simulink model "Speed_Controller_Test_gr2"  (Simulink 7.0)
settings: Solver=ode4  SolverMode=SingleTasking  StartTime=0.0  StopTime=252  FixedStep=0.01  RelTol=1e-3
InitFcn:
  | tempomat_para
StopFcn:
  | clear;
values from neighbouring files (symbols this model uses):
  A = 1.9    [tempomat_para.m]
  a_Fzg_max = 2    [tempomat_para.m]
  a_Fzg_min = -2    [tempomat_para.m]
  cw = 0.32    [tempomat_para.m]
  gang = [1 2 3 4]    [tempomat_para.m]
  gang_vec = [1 2 3 4]    [tempomat_para.m]
  i_anteil = 5    [tempomat_para.m]
  i_d = 3.42    [tempomat_para.m]
  i_g = [3.91 2.17 1.37 1.00]    [tempomat_para.m]
  lambda_gang = [1.3 1.25  1.17  1.05]    [tempomat_para.m]
  m_Fzg = 1400    [tempomat_para.m]
  M_mot_max = [130 149 163 170 168 166 162 158 150 139 123 80]    [tempomat_para.m]
  M_mot_min = [0 -40]    [tempomat_para.m]
  n_mot0 = 1000    [tempomat_para.m]
  n_mot_max = 1000:500:6500    [tempomat_para.m]
  n_mot_min = [1000 6500]    [tempomat_para.m]
  p_anteil = 100    [tempomat_para.m]
  r_dyn = 0.28    [tempomat_para.m]
  rho = 1.202    [tempomat_para.m]
  t_sch = 0.2    [tempomat_para.m]
  TI = [block '/TI']    [PSTI_callback.m]
  v_Fzg_ms0 = 0    [tempomat_para.m]
undefined symbols (not defined in the file or in its folder): Drossel_mat, getdatatypespecs
libraries: simulink x116, fzgbib x3
(part 1 of 10)
settings Model: Creator=Abel  LastModifiedBy=jza
settings DataIOCC: LimitDataPoints=off  SignalLoggingName=sigsOut
settings OptimizationCC: BooleanDataType=off
settings DebuggingCC: SaveWithParameterizedLinksMsg=none  SignalResolutionControl=TryResolveAllWithWarning  InheritedTsInSrcMsg=none  MultiTaskDSMMsg=warning  MultiTaskCondExecSysMsg=none  StrictBusMsg=None
settings RTWCC: IncludeERTFirstTime=on
settings GRTTargetCC: TargetFcnLib=ansi_tfl_tmw.mat

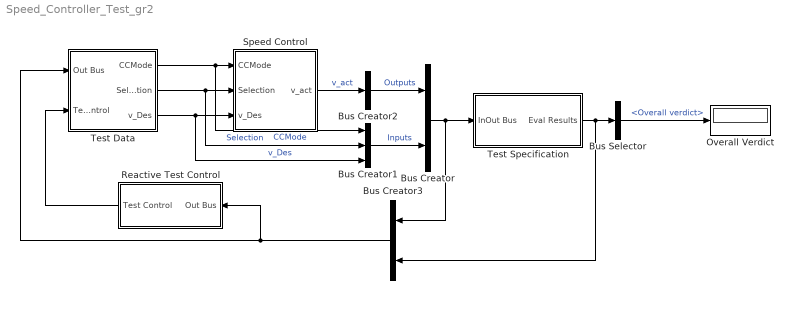
== system Speed_Controller_Test_gr2 ==
  Bus Creator : BusCreator  Inputs=2
  Bus Creator1 : BusCreator  Inputs=3
  Bus Creator2 : BusCreator  Inputs=1
  Bus Creator3 : BusCreator  Orientation=left  Inputs=2
  Bus Selector : BusSelector  OutputSignals=Overall verdict
  Overall Verdict : Display
  Reactive Test Control : Subsystem  Orientation=left
  Speed Control : Subsystem
  Test Data : Subsystem
  Test Specification : Subsystem  Description=Test evaluation system template. Create a new test evaluation system from this template.
  wires:
  Speed Control/1(v_act) -> Bus Creator2/1  "v_act"
  Bus Creator/1 -> Test Specification/1(InOut Bus), Bus Creator3/1
  Bus Creator2/1 -> Bus Creator/1  "Outputs"
  Bus Creator1/1 -> Bus Creator/2  "Inputs"
  Test Data/3(v_Des) -> Speed Control/3(v_Des), Bus Creator1/3  "v_Des"
  Bus Creator3/1 -> Test Data/1(Out Bus), Reactive Test Control/1(Out Bus)
  Test Specification/1(Eval Results) -> Bus Creator3/2, Bus Selector/1
  Reactive Test Control/1(Test Control) -> Test Data/2(Test Control)
  Bus Selector/1 -> Overall Verdict/1  "<Overall verdict>"
  Test Data/1(CCMode) -> Speed Control/1(CCMode), Bus Creator1/1  "CCMode"
  Test Data/2(Selection) -> Speed Control/2(Selection), Bus Creator1/2  "Selection"

== system Speed_Controller_Test_gr2/Reactive Test Control ==
  Out Bus : Inport  OutDataType=sfix(16)  OutScaling=2^0
  Bus Selector : BusSelector  OutputSignals=signal2.signal1.signal1.signal1.signal1.Local verdict
  Counter : Subsystem
  Memory : Memory
  OR : Logic  Operator=OR  Inputs=3  AllPortsSameDT=off  OutDataTypeMode=boolean
  Switch : Switch  Criteria=u2 > Threshold
  error : simulink/Logic and Bit Operations/Compare To Constant  SystemSampleTime=-1  relop===  const=-1  LogicOutDataTypeMode=uint8  ZeroCross=off
  fail : simulink/Logic and Bit Operations/Compare To Constant  SystemSampleTime=-1  relop===  const=0  LogicOutDataTypeMode=uint8  ZeroCross=off
  pass : simulink/Logic and Bit Operations/Compare To Constant  SystemSampleTime=-1  relop===  const=1  LogicOutDataTypeMode=uint8  ZeroCross=off
  test case 1 : Constant  OutDataType=sfix(16)  OutScaling=2^0
  test case 2 : Constant  Value=2  OutDataType=sfix(16)  OutScaling=2^0
  Test Control : Outport  OutDataType=sfix(16)  OutScaling=2^0
  wires:
  OR/1 -> Counter/1(In1), Counter/Trigger
  test case 1/1 -> Switch/3
  Out Bus/1 -> Bus Selector/1
  Switch/1 -> Test Control/1
  test case 2/1 -> Switch/1
  Counter/1(Out1) -> Switch/2
  Bus Selector/1 -> Memory/1  "<Local verdict>"
  pass/1 -> OR/1
  fail/1 -> OR/2
  error/1 -> OR/3
  Memory/1 -> pass/1, error/1, fail/1

== system Speed_Controller_Test_gr2/Speed Control ==
  CCMode : Inport  OutDataType=sfix(16)  OutScaling=2^0
  Selection : Inport  Port=2  OutDataType=sfix(16)  OutScaling=2^0
  v_Des : Inport  Port=3  OutDataType=sfix(16)  OutScaling=2^0
  " Speed Controller " : Subsystem  AncestorBlock=fzgbib/GeschwindigkeitsRegelung
  Terminator1 : Terminator
  Terminator2 : Terminator
  Vehicle Model : Subsystem
      mask Type: Vehicle Model
      mask Display: image(imread('car.jpg','jpg'),[0.05,0.2,0.9,0.6])
  v_act : Outport  OutDataType=sfix(16)  OutScaling=2^0
  wires:
  Vehicle Model/2(M_Br_b) -> Terminator1/1
  Vehicle Model/3(M_Mot_b) -> Terminator2/1
  " Speed Controller "/1(CarInputs) -> Vehicle Model/1(StellgroessenTempomat)
  Vehicle Model/1(FzgDaten) -> " Speed Controller "/1(CarOutputs)
  " Speed Controller "/2(v_act) -> v_act/1
  v_Des/1 -> " Speed Controller "/2(CCMode)
  Selection/1 -> " Speed Controller "/3(Selection)
  CCMode/1 -> " Speed Controller "/4(v_Des)

== system Speed_Controller_Test_gr2/Test Data ==
  Out Bus : Inport  OutDataType=sfix(16)  OutScaling=2^0
  Test Control : Inport  Port=2  OutDataType=sfix(16)  OutScaling=2^0
  Bus Creator : BusCreator  Inputs=6
  Bus Selector : BusSelector  OutputSignals=v_Des (signal 1),v_Des (signal 4)
  Bus Selector1 : BusSelector  OutputSignals=CCMode (signal 2),CCMode (signal 5)
  Bus Selector2 : BusSelector  OutputSignals=Selection (signal 3),Selection (signal 6)
  PrecAct CCMode : MultiPortSwitch  Inputs=3  zeroidx=on
  PrecAct Selection : MultiPortSwitch  Inputs=3  zeroidx=on
  PrecAct v_Des : MultiPortSwitch  Inputs=3  zeroidx=on
  R1 Speed Control step response : Subsystem
  R2 Speed Control velocity restoration time after simple  acceleration/deceleration : Subsystem
  zero signal : Constant  Value=0  OutDataType=sfix(16)  OutScaling=2^0
  CCMode : Outport  OutDataType=sfix(16)  OutScaling=2^0
  Selection : Outport  Port=2  OutDataType=sfix(16)  OutScaling=2^0
  v_Des : Outport  Port=3  OutDataType=sfix(16)  OutScaling=2^0
  wires:
  Out Bus/1 -> R1 Speed Control step response/1(Out Bus)
  PrecAct v_Des/1 -> v_Des/1
  zero signal/1 -> PrecAct v_Des/2, PrecAct Selection/2, PrecAct CCMode/2
  PrecAct CCMode/1 -> CCMode/1
  PrecAct Selection/1 -> Selection/1
  Bus Creator/1 -> Bus Selector/1, Bus Selector1/1, Bus Selector2/1
  Bus Selector/1 -> PrecAct v_Des/3  "<v_Des (signal 1)>"
  R1 Speed Control step response/1(v_Des) -> Bus Creator/1
  R1 Speed Control step response/2(CCMode) -> Bus Creator/2
  R1 Speed Control step response/3(Selection) -> Bus Creator/3
  R2 Speed Control velocity restoration time after simple  acceleration/deceleration/1(v_Des) -> Bus Creator/4
  R2 Speed Control velocity restoration time after simple  acceleration/deceleration/2(CCMode) -> Bus Creator/5
  R2 Speed Control velocity restoration time after simple  acceleration/deceleration/3(Selection) -> Bus Creator/6
  Bus Selector/2 -> PrecAct v_Des/4  "<v_Des (signal 4)>"
  Bus Selector1/1 -> PrecAct CCMode/3  "<CCMode (signal 2)>"
  Bus Selector1/2 -> PrecAct CCMode/4  "<CCMode (signal 5)>"
  Bus Selector2/1 -> PrecAct Selection/3  "<Selection (signal 3)>"
  Bus Selector2/2 -> PrecAct Selection/4  "<Selection (signal 6)>"
  Test Control/1 -> PrecAct v_Des/1, PrecAct CCMode/1, PrecAct Selection/1

== system Speed_Controller_Test_gr2/Test Specification ==
  InOut Bus : Inport  OutDataType=sfix(16)  OutScaling=2^0
  Arbitration : Subsystem
  Bus Creator1 : BusCreator  Inputs=2
  Bus Creator2 : BusCreator  Inputs=2
  Bus Selector1 : BusSelector  OutputSignals=signal1.signal1.signal1.Local verdict,signal1.signal1.signal2.Local verdict,signal2.signal1.signal1.Local verdict
  R1 Speed Control step response : Subsystem  Description=Requirement template. Create a new requirement from this template.
  R2 Speed Control velocity restoration time after simple  acceleration/deceleration : Subsystem  Description=Requirement template. Create a new requirement from this template.
  Signal Conversion : SignalConversion  ConversionOutput=Bus copy
  Eval Results : Outport  OutDataType=sfix(16)  OutScaling=2^0
  wires:
  Signal Conversion/1 -> R1 Speed Control step response/1(InOut Bus), R2 Speed Control velocity restoration time after simple  acceleration/deceleration/1(InOut Bus)
  R1 Speed Control step response/1(Test Info) -> Bus Creator2/1
  InOut Bus/1 -> Signal Conversion/1
  Bus Creator2/1 -> Bus Selector1/1, Bus Creator1/1
  R2 Speed Control velocity restoration time after simple  acceleration/deceleration/1(Test Info) -> Bus Creator2/2
  Bus Selector1/1 -> Arbitration/1(In1)  "<Local verdict>"
  Bus Selector1/2 -> Arbitration/2(In2)  "<Local verdict>"
  Bus Selector1/3 -> Arbitration/3(In3)  "<Local verdict>"
  Bus Creator1/1 -> Eval Results/1
  Arbitration/1(Out1) -> Bus Creator1/2  "Overall verdict"

== system Speed_Controller_Test_gr2/Reactive Test Control/Counter ==
  In1 : Inport  OutDataType=sfix(16)  OutScaling=2^0
  Trigger : TriggerPort
  " 1" : DataTypeConversion  Orientation=down  OutDataType=sfix(16)  OutScaling=2^0
  Add : Sum  OutDataType=sfix(16)  OutScaling=2^-10
  Memory : Memory  Orientation=left  InheritSampleTime=on
  Number of triggers : Constant  Value=2  OutDataType=sfix(16)  OutScaling=2^0
  Relational Operator1 : RelationalOperator  Operator===  LogicOutDataTypeMode=boolean
  Scope1 : Scope  NumInputPorts=4
      settings: YMin=182.932~-5~-5~-5  YMax=202.188~5~5~5  SaveName=ScopeData14  MaxDataPoints=5000000
  Out1 : Outport  OutDataType=sfix(16)  OutScaling=2^0
  wires:
  In1/1 -> Add/1, Scope1/2
  Number of triggers/1 -> Relational Operator1/2
  Relational Operator1/1 -> Out1/1
  Add/1 -> " 1"/1, Relational Operator1/1, Scope1/3
  Memory/1 -> Add/2
  " 1"/1 -> Memory/1

== system Speed_Controller_Test_gr2/Speed Control/ Speed Controller  ==
  CarOutputs : Inport  OutDataType=sfix(16)  OutScaling=2^0
  CCMode : Inport  Port=2  OutDataType=sfix(16)  OutScaling=2^0
  Selection : Inport  Port=3  OutDataType=sfix(16)  OutScaling=2^0
  v_Des : Inport  Port=4  OutDataType=sfix(16)  OutScaling=2^0
  Bus Selector : BusSelector  OutputSignals=i_Total,n_Eng,a_Vhcl,v_act
  Compute SUC inputs : Subsystem  AncestorBlock=fzgbib/StellgroessenBerechnung BeschleunigungsBegrenzung
  Speed Controller : Subsystem  AncestorBlock=fzgbib/GeschwindigkeitsRegelung
  "km/h -> m/s2" : Gain  Gain=1/3.6  ParameterDataType=sfix(16)  ParameterScaling=2^0  OutDataType=sfix(16)  OutScaling=2^0  SaturateOnIntegerOverflow=on
  "m/s2 -> km/h" : Gain  Gain=3.6  ParameterDataType=sfix(16)  ParameterScaling=2^0  OutDataType=sfix(16)  OutScaling=2^0  SaturateOnIntegerOverflow=on
  CarInputs : Outport  OutDataType=sfix(16)  OutScaling=2^0
  v_act : Outport  Port=2  OutDataType=sfix(16)  OutScaling=2^0
  wires:
  Speed Controller/1(T) -> Compute SUC inputs/4(T)
  Bus Selector/1 -> Compute SUC inputs/1(i_Total)  "<i_Total>"
  Bus Selector/2 -> Compute SUC inputs/2(n_Eng)  "<n_Eng>"
  Bus Selector/3 -> Compute SUC inputs/3(a_Vhcl)  "<a_Vhcl>"
  Bus Selector/4 -> Speed Controller/1(v_Vhcl), "m/s2 -> km/h"/1  "<v_act>"
  Compute SUC inputs/1(SUC inputs) -> CarInputs/1
  v_Des/1 -> "km/h -> m/s2"/1
  "km/h -> m/s2"/1 -> Speed Controller/2(v_Des)
  Selection/1 -> Speed Controller/3(Selection)
  CCMode/1 -> Speed Controller/4(CCMode)
  CarOutputs/1 -> Bus Selector/1
  "m/s2 -> km/h"/1 -> v_act/1

== system Speed_Controller_Test_gr2/Speed Control/Vehicle Model ==
  note: i_Gesamt
      | n_mot
      | a_Fzg_mss
      | v_Fzg_ms
      | Gang_i
  StellgroessenTempomat : Inport  Orientation=left  OutDataType=sfix(16)  OutScaling=2^0
  Bremsmomenten beschaenkung : fzgbib/Bremsmomenten beschraenkung  Orientation=left  SystemSampleTime=-1
  Bus Creator : BusCreator  Orientation=left  Inputs=5
  Const : Constant  OutDataType=sfix(16)  OutScaling=2^0
  Fahrzeugmodell : Subsystem  Orientation=left  AncestorBlock=fzgbib/Fahrzeugmodell
  Gangberechnung : fzgbib/Gangberechnung  Orientation=left  SystemSampleTime=-1
  M_Mot M_Br : Demux  Orientation=left  Outputs=2
  Motormoment beschraenkung : fzgbib/Motormoment beschraenkung  Orientation=left  SystemSampleTime=-1
  SG-Koordinator : Subsystem  Orientation=left
  Terminator : Terminator
  FzgDaten : Outport  Orientation=left  OutDataType=sfix(16)  OutScaling=2^0
  M_Br_b : Outport  Orientation=left  Port=2  OutDataType=sfix(16)  OutScaling=2^0
  M_Mot_b : Outport  Orientation=left  Port=3  OutDataType=sfix(16)  OutScaling=2^0
  wires:
  M_Mot M_Br/1 -> Gangberechnung/1, Motormoment beschraenkung/1
  Fahrzeugmodell/5(a_Fzg_mss) -> Bus Creator/3  "a_Vhcl"
  Fahrzeugmodell/1(v_Fzg_ms) -> Bus Creator/4  "v_act"
  Motormoment beschraenkung/1 -> Fahrzeugmodell/2(M_Mot_b), M_Mot_b/1
  M_Mot M_Br/2 -> Bremsmomenten beschaenkung/1
  Fahrzeugmodell/4(Gang_i) -> Gangberechnung/3, Bus Creator/5  "Gang_i"
  Fahrzeugmodell/6("DK_Stellung ") -> Terminator/1
  Fahrzeugmodell/3(n_Mot) -> Gangberechnung/2, Motormoment beschraenkung/2, Bus Creator/2  "n_Eng"
  Fahrzeugmodell/2(i_gesamt) -> Bus Creator/1  "i_Total"
  Gangberechnung/1 -> Fahrzeugmodell/3(Gang_w)
  SG-Koordinator/1(Momente) -> M_Mot M_Br/1
  Bremsmomenten beschaenkung/1 -> Fahrzeugmodell/1(M_Br_b), M_Br_b/1
  StellgroessenTempomat/1 -> SG-Koordinator/1(Tempomat), SG-Koordinator/3(Fahrer)
  Const/1 -> SG-Koordinator/2(TempomatFlag)
  Bus Creator/1 -> FzgDaten/1

== system Speed_Controller_Test_gr2/Test Data/R1 Speed Control step response ==
  Out Bus : Inport  OutDataType=sfix(16)  OutScaling=2^0
  Complete step & CC active + no target & Speed Control active : Subsystem  Description=Preconditions template. Create new preconditions blocks using this template.
  v_Des : Outport  OutDataType=sfix(16)  OutScaling=2^0
  CCMode : Outport  Port=2  OutDataType=sfix(16)  OutScaling=2^0
  Selection : Outport  Port=3  OutDataType=sfix(16)  OutScaling=2^0
  wires:
  Complete step & CC active + no target & Speed Control active/1(v_Des) -> v_Des/1  "v_Des"
  Complete step & CC active + no target & Speed Control active/2(CCMode) -> CCMode/1  "CCMode"
  Complete step & CC active + no target & Speed Control active/3(Selection) -> Selection/1  "Selection"
  Out Bus/1 -> Complete step & CC active + no target & Speed Control active/1(Out Bus)

== system Speed_Controller_Test_gr2/Test Data/R2 Speed Control velocity restoration time after simple  acceleration/deceleration ==
  " CC active + no target & Speed Control active & V_Des increases/decreases  7 times by 1 unit" : Subsystem  Description=Preconditions template. Create new preconditions blocks using this template.
  v_Des : Outport  OutDataType=sfix(16)  OutScaling=2^0
  CCMode : Outport  Port=2  OutDataType=sfix(16)  OutScaling=2^0
  Selection : Outport  Port=3  OutDataType=sfix(16)  OutScaling=2^0
  wires:
  " CC active + no target & Speed Control active & V_Des increases/decreases  7 times by 1 unit"/2(CCMode) -> CCMode/1  "CCMode"
  " CC active + no target & Speed Control active & V_Des increases/decreases  7 times by 1 unit"/3(Selection) -> Selection/1  "Selection"
  " CC active + no target & Speed Control active & V_Des increases/decreases  7 times by 1 unit"/1(v_Des) -> v_Des/1  "v_Des"

== system Speed_Controller_Test_gr2/Test Specification/Arbitration ==
  In1 : Inport  OutDataType=sfix(16)  OutScaling=2^0
  In2 : Inport  Port=2  OutDataType=sfix(16)  OutScaling=2^0
  In3 : Inport  Port=3  OutDataType=sfix(16)  OutScaling=2^0
  Collect Verdicts : MinMax  Inputs=4  OutDataType=sfix(16)  OutScaling=2^0
  Memory : Memory  Orientation=left  X0=2
  Out1 : Outport  OutDataType=sfix(16)  OutScaling=2^0
  wires:
  Memory/1 -> Collect Verdicts/4
  Collect Verdicts/1 -> Out1/1, Memory/1
  In1/1 -> Collect Verdicts/1
  In2/1 -> Collect Verdicts/2
  In3/1 -> Collect Verdicts/3

== system Speed_Controller_Test_gr2/Test Specification/R1 Speed Control step response ==
  InOut Bus : Inport  OutDataType=sfix(16)  OutScaling=2^0
  Bus Creator : BusCreator  Inputs=2
  Complete step & CC active + no target & Speed Control active : Subsystem  Description=Preconditions template. Create new preconditions blocks using this template.
  Maximum overshoot < 5 &  Steady state error < 5 : Subsystem  Description=Assertions template. Create a new assertions block from this template.
  Test Info : Outport  OutDataType=sfix(16)  OutScaling=2^0
  wires:
  InOut Bus/1 -> Complete step & CC active + no target & Speed Control active/1(InOut Bus), Maximum overshoot < 5 &  Steady state error < 5/2(InOut Bus)
  Maximum overshoot < 5 &  Steady state error < 5/1(VF info) -> Bus Creator/1
  Bus Creator/1 -> Test Info/1
  Complete step & CC active + no target & Speed Control active/1(Activate) -> Maximum overshoot < 5 &  Steady state error < 5/1(Precond), Bus Creator/2

== system Speed_Controller_Test_gr2/Test Specification/R2 Speed Control velocity restoration time after simple  acceleration/deceleration ==
  InOut Bus : Inport  OutDataType=sfix(16)  OutScaling=2^0
  Bus Creator : BusCreator  Inputs=2
  CC active + no target & Speed Control active & step of V_Des = |1|  with time periods >= 7s : Subsystem  Description=Preconditions template. Create new preconditions blocks using this template.
  after (6 seconds)  |V_Des-V_Vhcl <= 1.4| : Subsystem  Description=Assertions template. Create a new assertions block from this template.
  Test Info : Outport  OutDataType=sfix(16)  OutScaling=2^0
  wires:
  InOut Bus/1 -> CC active + no target & Speed Control active & step of V_Des = |1|  with time periods >= 7s/1(InOut Bus), after (6 seconds)  |V_Des-V_Vhcl <= 1.4|/2(InOut Bus)
  after (6 seconds)  |V_Des-V_Vhcl <= 1.4|/1(VF info) -> Bus Creator/1
  Bus Creator/1 -> Test Info/1
  CC active + no target & Speed Control active & step of V_Des = |1|  with time periods >= 7s/1(Activate) -> after (6 seconds)  |V_Des-V_Vhcl <= 1.4|/1(Precond), Bus Creator/2

== system Speed_Controller_Test_gr2/Speed Control/ Speed Controller /Compute SUC inputs ==
  note: M_Abtr_w_Temp [Nm]
      | (Abtriebswunschmoment _Tempomat)
  note: n_Mot [1/min]
      | (Motordrehzahl)
  note: a_Fzg [m/ss]
      | (Fzg.beschleunigung)
  i_Total : Inport  OutDataType=sfix(16)  OutScaling=2^0
  n_Eng : Inport  Port=2  OutDataType=sfix(16)  OutScaling=2^0
  a_Vhcl : Inport  Port=3  OutDataType=sfix(16)  OutScaling=2^0
  T : Inport  Port=4  OutDataType=sfix(16)  OutScaling=2^0
  Constant1 : Constant  Value=0  OutDataType=sfix(16)  OutScaling=2^0
  Gain : Gain  Gain=-1  ParameterDataType=sfix(16)  ParameterScaling=2^0  OutDataType=sfix(16)  OutScaling=2^0  SaturateOnIntegerOverflow=on
  Logical Operator : Logic  Operator=NOT  Inputs=1
  Mux : Mux  Inputs=2
  Oneway-Filter : Subsystem  mask(Oneway Filter){zk=2}
      mask prompts: zk "Filterkonstante"
      mask help: Filtert Signal mit Zeitkonstante zk nur, wenn kein Sprung auf Null von oben.
      mask Display: plot(0,0,100,100,[0 10 20 30 40 50 60 60 100],[0 0 30 50 60 65 67 0 0])
  Product : Product  Inputs=*/  OutDataType=sfix(16)  OutScaling=2^0  SaturateOnIntegerOverflow=on  InputSameDT=on
  Relational Operator : RelationalOperator  InputSameDT=on
  Saturation : Saturate  UpperLimit=m_Fzg*a_Fzg_max*r_dyn  LowerLimit=m_Fzg*a_Fzg_min*r_dyn
  Schleppmoment : Lookup  InputValues=n_mot_min  Table=M_mot_min  OutDataType=sfix(16)  OutScaling=2^0  SaturateOnIntegerOverflow=on
  Sum : Sum  OutDataType=sfix(16)  OutScaling=2^0  SaturateOnIntegerOverflow=on  InputSameDT=on
  Switch : Switch  Threshold=0.5  SaturateOnIntegerOverflow=on  InputSameDT=on
  Switch1 : Switch  Threshold=0.5  SaturateOnIntegerOverflow=on  InputSameDT=on
  neg_Beschleunigungsbegrenzung : Subsystem
  pos_Beschleunigungsbegrenzung : Subsystem
  SUC inputs : Outport  OutDataType=sfix(16)  OutScaling=2^0  InitialOutput=0
  wires:
  Schleppmoment/1 -> Relational Operator/2, Sum/1, Switch/3
  Relational Operator/1 -> Logical Operator/1, Switch/2
  Constant1/1 -> Switch1/3
  Logical Operator/1 -> Switch1/2
  Mux/1 -> SUC inputs/1
  neg_Beschleunigungsbegrenzung/1(M_Br3) -> Oneway-Filter/1(in)
  i_Total/1 -> Product/2
  Gain/1 -> Sum/2
  Sum/1 -> Switch1/1
  Switch/1 -> pos_Beschleunigungsbegrenzung/1(M_Mot_v)
  pos_Beschleunigungsbegrenzung/1(M_Mot3) -> Mux/1  "T_Engine"
  a_Vhcl/1 -> neg_Beschleunigungsbegrenzung/2(a_Fzg_mss), pos_Beschleunigungsbegrenzung/2(a_Fzg_mss)
  n_Eng/1 -> Schleppmoment/1, pos_Beschleunigungsbegrenzung/3("n_Mot ")
  Product/1 -> Relational Operator/1, Switch/1
  Switch1/1 -> neg_Beschleunigungsbegrenzung/1(M_Br_v)
  T/1 -> Saturation/1
  Saturation/1 -> Product/1, Gain/1
  Oneway-Filter/1("out ") -> neg_Beschleunigungsbegrenzung/3(M_Br_n), Mux/2  "T_Brake"

== system Speed_Controller_Test_gr2/Speed Control/ Speed Controller /Speed Controller ==
  note: v_soll [m/s] (Sollgeschw.)
  note: v_Fzg [m/s] (Istgeschw.)
  note: M_Abtr_w_GR [Nm]
      | (Abtriebswunschmoment _GR)
  v_Vhcl : Inport  OutDataType=sfix(16)  OutScaling=2^0
  v_Des : Inport  Port=2  OutDataType=sfix(16)  OutScaling=2^0
  Selection : Inport  Port=3  OutDataType=sfix(16)  OutScaling=2^0
  CCMode : Inport  Port=4  OutDataType=sfix(16)  OutScaling=2^0
  Constant : Constant  Value=0  OutDataType=sfix(16)  OutScaling=2^0
  Fcn2 : Fcn  Expr=u==2
  Fcn3 : Fcn  Expr=u!=ueberdrueckt
  Logical Operator : Logic
  Regler : Subsystem
  Stoergroessenkompensation : Subsystem
  Sum : Sum  Inputs=+-  OutDataType=sfix(16)  OutScaling=2^0  SaturateOnIntegerOverflow=on  InputSameDT=on
  Sum2 : Sum  Inputs=2  OutDataType=sfix(16)  OutScaling=2^0  SaturateOnIntegerOverflow=on  InputSameDT=on
  Switch : Switch  Threshold=0.5  SaturateOnIntegerOverflow=on  InputSameDT=on
  Switch1 : Switch  Threshold=0.5  SaturateOnIntegerOverflow=on  InputSameDT=on
  T : Outport  OutDataType=sfix(16)  OutScaling=2^0  InitialOutput=0
  wires:
  Logical Operator/1 -> Stoergroessenkompensation/3(GR_aktiv_l)
  Regler/1("u_R ") -> Sum2/2
  Stoergroessenkompensation/1(u_s) -> Sum2/1
  v_Vhcl/1 -> Stoergroessenkompensation/1(v_Fzg), Switch1/1
  Sum/1 -> Regler/1(d_v)
  Constant/1 -> Switch/3
  Switch1/1 -> Sum/2
  Fcn2/1 -> Logical Operator/1
  Selection/1 -> Fcn2/1
  CCMode/1 -> Fcn3/1
  Fcn3/1 -> Logical Operator/2, Switch1/2, Switch/2
  Switch/1 -> T/1
  Sum2/1 -> Switch/1
  v_Des/1 -> Switch1/3, Sum/1, Stoergroessenkompensation/2(v_soll)

== system Speed_Controller_Test_gr2/Speed Control/Vehicle Model/Fahrzeugmodell ==
  M_Br_b : Inport  OutDataType=sfix(16)  OutScaling=2^0
  M_Mot_b : Inport  Port=2  OutDataType=sfix(16)  OutScaling=2^0
  Gang_w : Inport  Port=3  OutDataType=sfix(16)  OutScaling=2^0
  Drosselklappenstellung : Subsystem
  Fahrwiderstaende : Subsystem
  Fahrzeugdynamik : Subsystem
  tw6 : ToWorkspace  VariableName=v_Fzg_kmh  SaveFormat=Array
      settings: MaxDataPoints=speicher
  v_Fzg_ms : Outport  OutDataType=sfix(16)  OutScaling=2^0  InitialOutput=0
  i_gesamt : Outport  Port=2  OutDataType=sfix(16)  OutScaling=2^0  InitialOutput=0
  n_Mot : Outport  Port=3  OutDataType=sfix(16)  OutScaling=2^0  InitialOutput=0
  Gang_i : Outport  Port=4  OutDataType=sfix(16)  OutScaling=2^0  InitialOutput=0
  a_Fzg_mss : Outport  Port=5  OutDataType=sfix(16)  OutScaling=2^0  InitialOutput=0
  "DK_Stellung " : Outport  Port=6  OutDataType=sfix(16)  OutScaling=2^0  InitialOutput=0
  wires:
  Fahrwiderstaende/7(schalt_l) -> Drosselklappenstellung/3(schalt_l)
  Fahrzeugdynamik/4(a_Fzg_mss) -> a_Fzg_mss/1
  Fahrzeugdynamik/1(v_Fzg_kmh) -> tw6/1
  Fahrwiderstaende/6(Gang_i) -> Gang_i/1, Fahrzeugdynamik/6(Gang_i)
  Fahrzeugdynamik/3(n_Mot) -> Drosselklappenstellung/1(n_mot), n_Mot/1
  Fahrzeugdynamik/2(v_Fzg_ms) -> Fahrwiderstaende/4(v_Fzg_ms), v_Fzg_ms/1
  Drosselklappenstellung/1(DK_Stellung [Grad]) -> "DK_Stellung "/1
  Fahrwiderstaende/1(F_A) -> Fahrzeugdynamik/1(F_A)
  Fahrwiderstaende/4(F_Brems) -> Fahrzeugdynamik/4(F_Brems)
  Fahrwiderstaende/2(F_L) -> Fahrzeugdynamik/2(F_L)
  Fahrwiderstaende/3(F_R) -> Fahrzeugdynamik/3(F_R)
  M_Mot_b/1 -> Drosselklappenstellung/2(M_Mot_b), Fahrwiderstaende/1(M_Mot_b)
  Gang_w/1 -> Fahrwiderstaende/3(Gang_w)
  M_Br_b/1 -> Fahrwiderstaende/2(M_Br_b)
  Fahrwiderstaende/5(i_gesamt) -> Fahrzeugdynamik/5(i_gesamt), i_gesamt/1

== system Speed_Controller_Test_gr2/Speed Control/Vehicle Model/SG-Koordinator ==
  note: TempomatFlag = 1 => Tempomat hat Priorität
  note: TempomatFlag = 0 => Fahrer hat Priorität
  Tempomat : Inport  OutDataType=sfix(16)  OutScaling=2^0
  TempomatFlag : Inport  Port=2  OutDataType=sfix(16)  OutScaling=2^0
  Fahrer : Inport  Port=3  OutDataType=sfix(16)  OutScaling=2^0
  Bus Selector : BusSelector  OutputSignals=T_Engine,T_Brake
  Bus Selector1 : BusSelector  OutputSignals=T_Engine,T_Brake
  Constant3 : Constant  OutDataType=sfix(16)  OutScaling=2^0
  Multiport Switch : MultiPortSwitch  Inputs=2  SaturateOnIntegerOverflow=on  InputSameDT=on
  Mux : Mux  Inputs=2
  Mux1 : Mux  Inputs=2
  Sum : Sum  OutDataType=sfix(16)  OutScaling=2^0  SaturateOnIntegerOverflow=on  InputSameDT=on
  Momente : Outport  OutDataType=sfix(16)  OutScaling=2^0  InitialOutput=0
  wires:
  Multiport Switch/1 -> Momente/1
  Sum/1 -> Multiport Switch/1
  Constant3/1 -> Sum/2
  TempomatFlag/1 -> Sum/1
  Bus Selector/1 -> Mux/1  "<T_Engine>"
  Bus Selector/2 -> Mux/2  "<T_Brake>"
  Tempomat/1 -> Bus Selector/1
  Mux/1 -> Multiport Switch/3
  Bus Selector1/1 -> Mux1/1  "<T_Engine>"
  Bus Selector1/2 -> Mux1/2  "<T_Brake>"
  Fahrer/1 -> Bus Selector1/1
  Mux1/1 -> Multiport Switch/2

== system Speed_Controller_Test_gr2/Test Data/R1 Speed Control step response/Complete step & CC active + no target & Speed Control active ==
  Out Bus : Inport  OutDataType=sfix(16)  OutScaling=2^0
  Active : Constant  Value=2  OutDataType=sfix(16)  OutScaling=2^0
  Active + no target : Constant  Value=2  OutDataType=sfix(16)  OutScaling=2^0
  Generate complete step : Subsystem  mask(Feature generation){XO=80, XF=100, t=60, size=-50, const=20}
      mask prompts: XO "Initial Value:"; XF "Final Value:"; t "Step Time:"; size "Second Step Size:"; const "Constant duration before step appears:"
      mask help: Complete step generation using trigger signal from VF: Step response characteristics.
      mask Display: plot([1,2,3,4,4.0001,6,7,7.0001,9,10],[1,1,1,1,4,4,4,2,2,2])
  v_Des : Outport  OutDataType=sfix(16)  OutScaling=2^0
  CCMode : Outport  Port=2  OutDataType=sfix(16)  OutScaling=2^0
  Selection : Outport  Port=3  OutDataType=sfix(16)  OutScaling=2^0
  wires:
  Out Bus/1 -> Generate complete step/1(Out Bus)
  Generate complete step/1(v_Des) -> v_Des/1
  Active + no target/1 -> CCMode/1
  Active/1 -> Selection/1

== system Speed_Controller_Test_gr2/Test Data/R2 Speed Control velocity restoration time after simple  acceleration/deceleration/ CC active + no target & Speed Control active & V_Des increases/decreases  7 times by 1 unit ==
  Active : Constant  Value=2  OutDataType=sfix(16)  OutScaling=2^0
  Active + no target : Constant  Value=2  OutDataType=sfix(16)  OutScaling=2^0
  V_Des increases/decreases  7 times by 1 unit : Subsystem  Description=Preconditions template. Create new preconditions blocks using this template.
  v_Des : Outport  OutDataType=sfix(16)  OutScaling=2^0
  CCMode : Outport  Port=2  OutDataType=sfix(16)  OutScaling=2^0
  Selection : Outport  Port=3  OutDataType=sfix(16)  OutScaling=2^0
  wires:
  Active + no target/1 -> CCMode/1
  Active/1 -> Selection/1
  V_Des increases/decreases  7 times by 1 unit/1(v_Des) -> v_Des/1

== system Speed_Controller_Test_gr2/Test Specification/R1 Speed Control step response/Complete step & CC active + no target & Speed Control active ==
  InOut Bus : Inport  OutDataType=sfix(16)  OutScaling=2^0
  Active : Constant  Value=2  OutDataType=sfix(16)  OutScaling=2^0
  Active + no target : Constant  Value=2  OutDataType=sfix(16)  OutScaling=2^0
  Bus Selector : BusSelector  OutputSignals=Inputs.v_Des,Outputs.v_act,Inputs.CCMode,Inputs.Selection
  CC active & no target : Subsystem  mask(Range - Gap Absolute Tolerance){GorR=Range, AbsoluteTolerance=0}
      mask prompts: GorR "Use range or gap"; AbsoluteTolerance "Absolute Tolerance"
      mask help: Check that a signal stays inside a range or outside a gap around a reference signal. Specify the range or the gap absolute to the reference signal.
      mask init:
      | if max(get_param(gcb,'GorR') == ' ') % Gap
      |     helpVariable1 = '~=';
      | else % Range
      |     helpVariable1 = '==';
      | end
      | set_param([gcb '/Relational Operator'],'Operator',helpVariable1);
      mask StyleString: popup(Range|Gap  ),edit
      mask Display:
      | port_label('output',1,'A');
      | port_label('input',1,'Sig');
      | port_label('input',2,'Ref');
      | text(0.40,0.53,'+');
      | text(0.415,0.46,'-');
      | text(0.5,0.5,num2str(AbsoluteTolerance));
      | text(0.05,0.5,helpVariable1);
  Complete step : Constant  OutDataType=sfix(16)  OutScaling=2^0
  Complete step detection : Subsystem  mask(Complete step detection){Param=0}
      mask prompts: Param "Mask Parameter 1:"
  PS : Subsystem  mask(Feature layer: preconditions synchronization){NoTI=2, NoTDD=0, NoTID=1, TIdel=[0  0], TDDdel=[]}
      mask prompts: NoTI "Time-independent features identifiable with or without a delay (TI)"; NoTDD "Triggered features identifiable with determinate delay or without a delay (TDD)"; NoTID "Triggered features identifiable with indeterminate delay (TID)"; TIdel "Time-independent features delays (in time steps). E.g. [0 1 0] for 3 features"; TDDdel "Triggered features delays (in time steps). E.g. [0 0] for 2 features"
      mask help: Use this block for synchronizing the precondition features. For changing the block inputs, use the parameters below. The output must be used for assertions activation.
      mask init:
      | PS_init(gcb);
      mask StyleString: popup(0|1|2|3|4|5|6|7|8|9),popup(0|1|2|3|4|5|6|7|8|9),popup(0|1|2|3|4|5|6|7|8|9),edit,edit
      mask CallbackString:
      | PSTI_callback(gcb);|PSTDD_callback(gcb);|PSTID_callback(gcb);|NoTI = str2double(get_param(gcb,'NoTI'));
      | TIdel = str2num(get_param(gcb,'TIdel'));
      | if NoTI ~= length(TIdel) && NoTI ~= 0
      |     error(['The number of delays entered (' num2str(length(TIdel)) ') does not correspond to the above specified number of time-independent features (' num2str(NoTI) ').']);
      | end|NoTDD = str2double(get_param(gcb,'NoTDD'));
      | TDDdel = str2num(get_param(gcb,'TDDdel'));
      | if NoTDD ~= length(TDDdel) && NoTDD ~= 0
      |     error(['The number of delays entered (' num2str(length(TDDdel)) ') does not correspond to the above specified number of triggered features with constant delay (' num2str(NoTDD) ').']);
      | end
  Range - Gap Absolute tolerance Precond : Subsystem  mask(Range - Gap Absolute Tolerance){GorR=Range, AbsoluteTolerance=0}
      mask prompts: GorR "Use range or gap"; AbsoluteTolerance "Absolute Tolerance"
      mask help: Check that a signal stays inside a range or outside a gap around a reference signal. Specify the range or the gap absolute to the reference signal.
      mask init:
      | if max(get_param(gcb,'GorR') == ' ') % Gap
      |     helpVariable1 = '~=';
      | else % Range
      |     helpVariable1 = '==';
      | end
      | set_param([gcb '/Relational Operator'],'Operator',helpVariable1);
      mask StyleString: popup(Range|Gap  ),edit
      mask Display:
      | port_label('output',1,'A');
      | port_label('input',1,'Sig');
      | port_label('input',2,'Ref');
      | text(0.40,0.53,'+');
      | text(0.415,0.46,'-');
      | text(0.5,0.5,num2str(AbsoluteTolerance));
      | text(0.05,0.5,helpVariable1);
  Speed control active : Subsystem  mask(Range - Gap Absolute Tolerance){GorR=Range, AbsoluteTolerance=0}
      mask prompts: GorR "Use range or gap"; AbsoluteTolerance "Absolute Tolerance"
      mask help: Check that a signal stays inside a range or outside a gap around a reference signal. Specify the range or the gap absolute to the reference signal.
      mask init:
      | if max(get_param(gcb,'GorR') == ' ') % Gap
      |     helpVariable1 = '~=';
      | else % Range
      |     helpVariable1 = '==';
      | end
      | set_param([gcb '/Relational Operator'],'Operator',helpVariable1);
      mask StyleString: popup(Range|Gap  ),edit
      mask Display:
      | port_label('output',1,'A');
      | port_label('input',1,'Sig');
      | port_label('input',2,'Ref');
      | text(0.40,0.53,'+');
      | text(0.415,0.46,'-');
      | text(0.5,0.5,num2str(AbsoluteTolerance));
      | text(0.05,0.5,helpVariable1);
  Activate : Outport  OutDataType=sfix(16)  OutScaling=2^0
  wires:
  Complete step detection/1(R) -> PS/1(R TID1)
  Complete step detection/2(T) -> PS/2(T TID1)
  Complete step detection/3(Complete step) -> Range - Gap Absolute tolerance Precond/1(Signal)
  Complete step/1 -> Range - Gap Absolute tolerance Precond/2(Reference)
  Range - Gap Absolute tolerance Precond/1(Activate) -> PS/3(A TID1)
  PS/1(Precond) -> Activate/1
  InOut Bus/1 -> Bus Selector/1
  Bus Selector/1 -> Complete step detection/1(Step)  "<v_Des>"
  Bus Selector/2 -> Complete step detection/2(Step response)  "<v_act>"
  Bus Selector/3 -> CC active & no target/1(Signal)  "<CCMode>"
  Active + no target/1 -> CC active & no target/2(Reference)
  CC active & no target/1(Activate) -> PS/4(A TI1)
  Active/1 -> Speed control active/2(Reference)
  Speed control active/1(Activate) -> PS/5(A TI2)
  Bus Selector/4 -> Speed control active/1(Signal)  "<Selection>"

== system Speed_Controller_Test_gr2/Test Specification/R1 Speed Control step response/Maximum overshoot < 5 &  Steady state error < 5 ==
  Precond : Inport  OutDataType=sfix(16)  OutScaling=2^0
  InOut Bus : Inport  Port=2  OutDataType=sfix(16)  OutScaling=2^0
  Abs : Abs
  Bus Creator : BusCreator  Inputs=2
  Bus Selector : BusSelector  OutputSignals=Inputs.v_Des,Outputs.v_act
  Maximum Overshoot : Constant  Value=5  OutDataType=sfix(16)  OutScaling=2^0
  Maximum overshoot < 5 : Subsystem  mask(Bound){cm=<, Lower=1, Upper=0, Ass=[1 2], Pre=[1 2], Req=[1 2]}
      mask prompts: cm "Comparison method:"; Upper "Mask Parameter 3:"; Req "Mask Parameter 6:"
      mask help:
      | Compare a signal with a reference using the specified comparison method.
      |
      | Output verdict V and lower (LL) and upper (UL) limits for reporting.
      |
      | For '==' or '~=' use "Range - Gap"
      mask init:
      | set_param([get_param(gcb,'Parent') '/' get_param(gcb,'Name') '/Relational Operator'],'Operator',get_param(gcb,'cm'));
      | set_param(gcb,'Upper',num2str(uint8(max(get_param([get_param(gcb,'Parent') '/' get_param(gcb,'Name') '/Relational Operator'],'Operator') == '>'))));
      | set_param(gcb,'Lower',num2str(uint8(max(get_param([get_param(gcb,'Parent') '/' get_param(gcb,'Name') '/Relational Operator'],'Operator') == '<'))));
      | set_param(gcb, ...
      |           'Ass', ...
      |           ['[1 2]']);
      | set_param(gcb, ...
      |           'Pre', ...
      |           ['[1 2]']); 
      | set_param(gcb, ...
      |           'Req', ...
      |           ['[1 2]']);
      mask StyleString: popup(>|>=|<=|<),edit,edit,edit,edit,edit
      mask Display:
      | port_label('output', 1, ['V']);
      | port_label('input', 1, 'Sig');
      | port_label('input', 2, 'Ref');
      | text(0.05,0.5,get_param(get_param([get_param(gcb,'Parent') '/' get_param(gcb,'Name') '/Relational Operator'],'handle'),'Operator'));
  PAS : Subsystem  mask{AFT=TID, AFD=2}
      mask prompts: AFT "Assertion feature type:"; AFD "Assertion feature delay (in time steps)"
      mask init:
      | PAS_init(gcb);
      mask StyleString: popup(TI|TDD|TID),edit
      mask CallbackString: PAS_callback(gcb);|
  PAS1 : Subsystem  mask{AFT=TID, AFD=2}
      mask prompts: AFT "Assertion feature type:"; AFD "Assertion feature delay (in time steps)"
      mask init:
      | PAS_init(gcb);
      mask StyleString: popup(TI|TDD|TID),edit
      mask CallbackString: PAS_callback(gcb);|
  Steady state error < 5 : Subsystem  mask(Bound){cm=<, Lower=1, Upper=0, Ass=[1 2], Pre=[1 2], Req=[1 2]}
      mask prompts: cm "Comparison method:"; Upper "Mask Parameter 3:"; Req "Mask Parameter 6:"
      mask help:
      | Compare a signal with a reference using the specified comparison method.
      |
      | Output verdict V and lower (LL) and upper (UL) limits for reporting.
      |
      | For '==' or '~=' use "Range - Gap"
      mask init: same as Speed_Controller_Test_gr2/Test Specification/R1 Speed Control step response/Maximum overshoot < 5 &  Steady state error < 5/Maximum overshoot < 5
      mask StyleString: popup(>|>=|<=|<),edit,edit,edit,edit,edit
      mask Display:
      | port_label('output', 1, ['V']);
      | port_label('input', 1, 'Sig');
      | port_label('input', 2, 'Ref');
      | text(0.05,0.5,get_param(get_param([get_param(gcb,'Parent') '/' get_param(gcb,'Name') '/Relational Operator'],'handle'),'Operator'));
  Steady state error : Constant  Value=5  OutDataType=sfix(16)  OutScaling=2^0
  Step response characteristics : Subsystem  mask(Step response characteristics){Param=0}
      mask prompts: Param "Mask Parameter 1:"
  Terminator{1..4} (4 alike) : Terminator
  VF info : Outport  OutDataType=sfix(16)  OutScaling=2^0
  wires:
  Bus Selector/1 -> Step response characteristics/1(Step)  "<v_Des>"
  Step response characteristics/1(R) -> PAS1/2(R), PAS/2(R)  "Ra"
  PAS/1(VF Info) -> Bus Creator/1
  Precond/1 -> PAS1/1(Precond), PAS/1(Precond)
  InOut Bus/1 -> Bus Selector/1
  Bus Creator/1 -> VF info/1
  Bus Selector/2 -> Step response characteristics/2(Step response)  "<v_act>"
  PAS1/1(VF Info) -> Bus Creator/2
  Maximum overshoot < 5/1(V) -> PAS/4(V)
  Maximum Overshoot/1 -> Maximum overshoot < 5/2(Reference)
  Step response characteristics/7(Maximum Overshoot) -> Abs/1
  Step response characteristics/3(Overshoot T) -> PAS/3(T)  "Ta"
  Step response characteristics/5(Steady state error T) -> PAS1/3(T)  "Ta"
  Steady state error < 5/1(V) -> PAS1/4(V)
  Steady state error/1 -> Steady state error < 5/2(Reference)
  Step response characteristics/9(Steady state error) -> Steady state error < 5/1(Signal)
  Step response characteristics/8(Settling time) -> Terminator4/1
  Step response characteristics/6(Rise time) -> Terminator3/1
  Step response characteristics/4(Settling time T) -> Terminator2/1
  Step response characteristics/2(Rise time T) -> Terminator1/1
  Abs/1 -> Maximum overshoot < 5/1(Signal)

== system Speed_Controller_Test_gr2/Test Specification/R2 Speed Control velocity restoration time after simple  acceleration/deceleration/CC active + no target & Speed Control active & step of V_Des = |1|  with time periods >= 7s ==
  InOut Bus : Inport  OutDataType=sfix(16)  OutScaling=2^0
  Active : Constant  Value=2  OutDataType=sfix(16)  OutScaling=2^0
  Active + no target : Constant  Value=2  OutDataType=sfix(16)  OutScaling=2^0
  Bus Selector : BusSelector  OutputSignals=Inputs.v_Des,Inputs.CCMode,Inputs.Selection
  CC active & no target : Subsystem  mask(Range - Gap Absolute Tolerance){GorR=Range, AbsoluteTolerance=0}
      mask prompts: GorR "Use range or gap"; AbsoluteTolerance "Absolute Tolerance"
      mask help: Check that a signal stays inside a range or outside a gap around a reference signal. Specify the range or the gap absolute to the reference signal.
      mask init:
      | if max(get_param(gcb,'GorR') == ' ') % Gap
      |     helpVariable1 = '~=';
      | else % Range
      |     helpVariable1 = '==';
      | end
      | set_param([gcb '/Relational Operator'],'Operator',helpVariable1);
      mask StyleString: popup(Range|Gap  ),edit
      mask Display:
      | port_label('output',1,'A');
      | port_label('input',1,'Sig');
      | port_label('input',2,'Ref');
      | text(0.40,0.53,'+');
      | text(0.415,0.46,'-');
      | text(0.5,0.5,num2str(AbsoluteTolerance));
      | text(0.05,0.5,helpVariable1);
  CC active & no target1 : Subsystem  mask(Range - Gap Absolute Tolerance){GorR=Range, AbsoluteTolerance=0}
      mask prompts: GorR "Use range or gap"; AbsoluteTolerance "Absolute Tolerance"
      mask help: Check that a signal stays inside a range or outside a gap around a reference signal. Specify the range or the gap absolute to the reference signal.
      mask init:
      | if max(get_param(gcb,'GorR') == ' ') % Gap
      |     helpVariable1 = '~=';
      | else % Range
      |     helpVariable1 = '==';
      | end
      | set_param([gcb '/Relational Operator'],'Operator',helpVariable1);
      mask StyleString: popup(Range|Gap  ),edit
      mask Display:
      | port_label('output',1,'A');
      | port_label('input',1,'Sig');
      | port_label('input',2,'Ref');
      | text(0.40,0.53,'+');
      | text(0.415,0.46,'-');
      | text(0.5,0.5,num2str(AbsoluteTolerance));
      | text(0.05,0.5,helpVariable1);
  PS : Subsystem  mask(Feature layer: preconditions synchronization){NoTI=3, NoTDD=0, NoTID=0, TIdel=[0  0  0], TDDdel=[]}
      mask prompts: NoTI "Time-independent features identifiable with or without a delay (TI)"; NoTDD "Triggered features identifiable with determinate delay or without a delay (TDD)"; NoTID "Triggered features identifiable with indeterminate delay (TID)"; TIdel "Time-independent features delays (in time steps). E.g. [0 1 0] for 3 features"; TDDdel "Triggered features delays (in time steps). E.g. [0 0] for 2 features"
      mask help: Use this block for synchronizing the precondition features. For changing the block inputs, use the parameters below. The output must be used for assertions activation.
      mask init:
      | PS_init(gcb);
      mask StyleString: popup(0|1|2|3|4|5|6|7|8|9),popup(0|1|2|3|4|5|6|7|8|9),popup(0|1|2|3|4|5|6|7|8|9),edit,edit
      mask CallbackString:
      | PSTI_callback(gcb);|PSTDD_callback(gcb);|PSTID_callback(gcb);|NoTI = str2double(get_param(gcb,'NoTI'));
      | TIdel = str2num(get_param(gcb,'TIdel'));
      | if NoTI ~= length(TIdel) && NoTI ~= 0
      |     error(['The number of delays entered (' num2str(length(TIdel)) ') does not correspond to the above specified number of time-independent features (' num2str(NoTI) ').']);
      | end|NoTDD = str2double(get_param(gcb,'NoTDD'));
      | TDDdel = str2num(get_param(gcb,'TDDdel'));
      | if NoTDD ~= length(TDDdel) && NoTDD ~= 0
      |     error(['The number of delays entered (' num2str(length(TDDdel)) ') does not correspond to the above specified number of triggered features with constant delay (' num2str(NoTDD) ').']);
      | end
  Scope1 : Scope  NumInputPorts=3
      settings: TimeRange=120  YMin=-0.003370786516853574~-5~-5  YMax=0.3966292134831465~5~5  SaveName=ScopeData5  MaxDataPoints=5000000
  Speed Control active : Subsystem  mask(Range - Gap Absolute Tolerance){GorR=Range, AbsoluteTolerance=0}
      mask prompts: GorR "Use range or gap"; AbsoluteTolerance "Absolute Tolerance"
      mask help: Check that a signal stays inside a range or outside a gap around a reference signal. Specify the range or the gap absolute to the reference signal.
      mask init:
      | if max(get_param(gcb,'GorR') == ' ') % Gap
      |     helpVariable1 = '~=';
      | else % Range
      |     helpVariable1 = '==';
      | end
      | set_param([gcb '/Relational Operator'],'Operator',helpVariable1);
      mask StyleString: popup(Range|Gap  ),edit
      mask Display:
      | port_label('output',1,'A');
      | port_label('input',1,'Sig');
      | port_label('input',2,'Ref');
      | text(0.40,0.53,'+');
      | text(0.415,0.46,'-');
      | text(0.5,0.5,num2str(AbsoluteTolerance));
      | text(0.05,0.5,helpVariable1);
  Step with step size=|1|  and time periods >= 6s detection : Subsystem  mask(Complete step detection){Param=0}
      mask prompts: Param "Mask Parameter 1:"
  true : Constant  OutDataType=sfix(16)  OutScaling=2^0
  Activate : Outport  OutDataType=sfix(16)  OutScaling=2^0
  wires:
  PS/1(Precond) -> Activate/1
  InOut Bus/1 -> Bus Selector/1
  Bus Selector/1 -> Step with step size=|1|  and time periods >= 6s detection/1(Step)  "<v_Des>"
  Bus Selector/2 -> CC active & no target/1(Signal)  "<CCMode>"
  Active + no target/1 -> CC active & no target/2(Reference)
  Active/1 -> Speed Control active/2(Reference)
  Bus Selector/3 -> Speed Control active/1(Signal)  "<Selection>"
  Step with step size=|1|  and time periods >= 6s detection/1(Complete step) -> CC active & no target1/1(Signal)
  true/1 -> CC active & no target1/2(Reference)
  CC active & no target1/1(Activate) -> PS/1(A TI1)
  CC active & no target/1(Activate) -> PS/2(A TI2)
  Speed Control active/1(Activate) -> PS/3(A TI3)

== system Speed_Controller_Test_gr2/Test Specification/R2 Speed Control velocity restoration time after simple  acceleration/deceleration/after (6 seconds)  |V_Des-V_Vhcl <= 1.4| ==
  Precond : Inport  OutDataType=sfix(16)  OutScaling=2^0
  InOut Bus : Inport  Port=2  OutDataType=sfix(16)  OutScaling=2^0
  " " : Subsystem  mask(Bound){cm=<=, Lower=1, Upper=0, Ass=[1 2], Pre=[1 2], Req=[1 2]}
      mask prompts: cm "Comparison method:"; Upper "Mask Parameter 3:"; Req "Mask Parameter 6:"
      mask help:
      | Compare a signal with a reference using the specified comparison method.
      |
      | Output verdict V and lower (LL) and upper (UL) limits for reporting.
      |
      | For '==' or '~=' use "Range - Gap"
      mask init: same as Speed_Controller_Test_gr2/Test Specification/R1 Speed Control step response/Maximum overshoot < 5 &  Steady state error < 5/Maximum overshoot < 5
      mask StyleString: popup(>|>=|<=|<),edit,edit,edit,edit,edit
      mask Display:
      | port_label('output', 1, ['V']);
      | port_label('input', 1, 'Sig');
      | port_label('input', 2, 'Ref');
      | text(0.05,0.5,get_param(get_param([get_param(gcb,'Parent') '/' get_param(gcb,'Name') '/Relational Operator'],'handle'),'Operator'));
  Bus Creator : BusCreator  Inputs=1
  Bus Selector : BusSelector  OutputSignals=Inputs.v_Des,Outputs.v_act
  Bus Selector{1..4} (4 alike) : BusSelector  OutputSignals=Local verdict
  PAS1 : Subsystem  mask{AFT=TI, AFD=600}
      mask prompts: AFT "Assertion feature type:"; AFD "Assertion feature delay (in time steps)"
      mask init:
      | PAS_init(gcb);
      mask StyleString: popup(TI|TDD|TID),edit
      mask CallbackString: PAS_callback(gcb);|
  PAS2 : Subsystem  mask{AFT=TI, AFD=600}
      mask prompts: AFT "Assertion feature type:"; AFD "Assertion feature delay (in time steps)"
      mask init:
      | PAS_init(gcb);
      mask StyleString: popup(TI|TDD|TID),edit
      mask CallbackString: PAS_callback(gcb);|
  R = 2 : Subsystem
  Scope : Scope  NumInputPorts=5
      settings: YMin=-5~-5~-5~80~0  YMax=5~5~5~107.5~110  SaveName=ScopeData2  MaxDataPoints=5000000
  t1 : Constant  Value=1.4  OutDataType=sfix(16)  OutScaling=2^0
  t2 : Constant  OutDataType=sfix(16)  OutScaling=2^0
  within(20 sec)1 : Subsystem  mask(Bound){cm=<=, Lower=1, Upper=0, Ass=[1 2], Pre=[1 2], Req=[1 2]}
      mask prompts: cm "Comparison method:"; Upper "Mask Parameter 3:"; Req "Mask Parameter 6:"
      mask help:
      | Compare a signal with a reference using the specified comparison method.
      |
      | Output verdict V and lower (LL) and upper (UL) limits for reporting.
      |
      | For '==' or '~=' use "Range - Gap"
      mask init: same as Speed_Controller_Test_gr2/Test Specification/R1 Speed Control step response/Maximum overshoot < 5 &  Steady state error < 5/Maximum overshoot < 5
      mask StyleString: popup(>|>=|<=|<),edit,edit,edit,edit,edit
      mask Display:
      | port_label('output', 1, ['V']);
      | port_label('input', 1, 'Sig');
      | port_label('input', 2, 'Ref');
      | text(0.05,0.5,get_param(get_param([get_param(gcb,'Parent') '/' get_param(gcb,'Name') '/Relational Operator'],'handle'),'Operator'));
  |V_Des-V_Vhcl| : Subsystem
  VF info : Outport  OutDataType=sfix(16)  OutScaling=2^0
  wires:
  t1/1 -> " "/2(Reference)
  " "/1(V) -> Bus Selector1/1, PAS1/2(V)
  InOut Bus/1 -> |V_Des-V_Vhcl|/1(InOut Bus), Bus Selector/1, R = 2/2(In2)
  Bus Creator/1 -> VF info/1
  Precond/1 -> PAS1/1(Precond), PAS2/1(Precond), R = 2/1(In1)
  PAS1/1(VF Info) -> Bus Creator/1, Bus Selector2/1
  |V_Des-V_Vhcl|/1(Out1) -> " "/1(Signal)
  t2/1 -> within(20 sec)1/2(Reference)
  within(20 sec)1/1(V) -> Bus Selector4/1, PAS2/2(V)
  R = 2/1(Out1) -> within(20 sec)1/1(Signal), Scope/3
  Bus Selector4/1 -> Scope/1  "<Local verdict>"
  PAS2/1(VF Info) -> Bus Selector3/1
  Bus Selector3/1 -> Scope/2  "<Local verdict>"
